simulink subsystem "As_Assembly"  (R2022b)
settings: Solver=VariableStepAuto  StartTime=0.0  StopTime=30  RelTol=1e-3
libraries: mbedblockslib x6, simulink x4, hdlsllib x2, slpidlib x2, fl_lib x1, nesl_utility x1
(part 3 of 3)

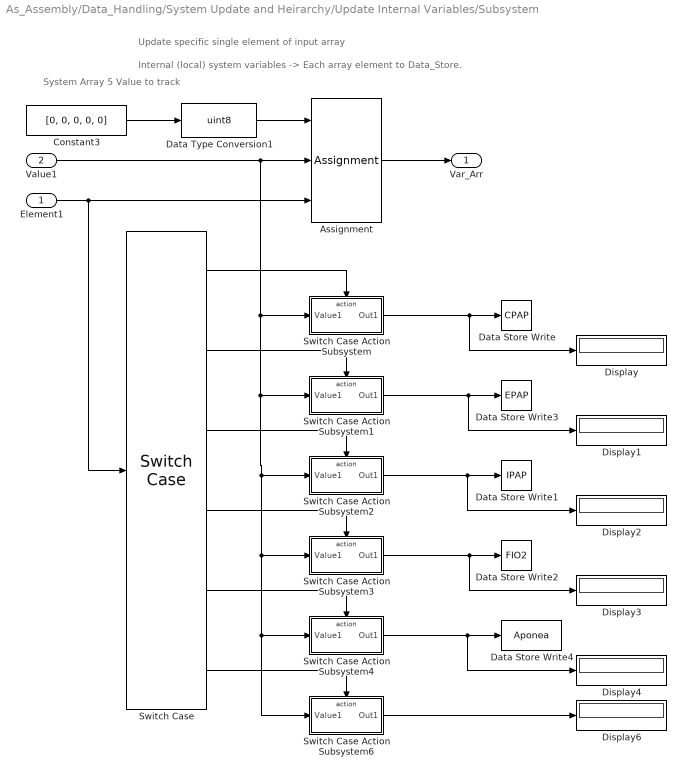
== system As_Assembly/Data_Handling/System Update and Heirarchy/Update Internal Variables/Subsystem ==
  note: System Array
      | 5 Value to track
  note: Update specific single element of input array
  note: Internal (local) system variables -> Each array element to Data_Store.
  Element1 : Inport
  Value1 : Inport  Port=2
  Assignment : Assignment  IndexMode=Zero-based  DiagnosticForDimensions=Warning  IndexOptions=Index vector (port)  Indices=0  OutputSizes=1
  Constant3 : Constant  Value=[0, 0, 0, 0, 0]
  Data Store Write : DataStoreWrite  DataStoreName=CPAP  IndexOptions=Index vector (dialog)  Indices=1  OutputSizes=1
  Data Store Write1 : DataStoreWrite  DataStoreName=IPAP  DataStoreElements=IPAP  IndexOptions=Index vector (dialog)  Indices=1  OutputSizes=1
  Data Store Write2 : DataStoreWrite  DataStoreName=FIO2  DataStoreElements=FIO2  IndexOptions=Index vector (dialog)  Indices=1  OutputSizes=1
  Data Store Write3 : DataStoreWrite  DataStoreName=EPAP  DataStoreElements=EPAP  IndexOptions=Index vector (dialog)  Indices=1  OutputSizes=1
  Data Store Write4 : DataStoreWrite  DataStoreName=Aponea  DataStoreElements=Aponea  IndexOptions=Index vector (dialog)  Indices=1  OutputSizes=1
  Data Type Conversion1 : DataTypeConversion  OutDataTypeStr=uint8  SaturateOnIntegerOverflow=off  RndMeth=Floor
  Display{,1..4,6} (6 alike) : Display
  Switch Case : SwitchCase  CaseConditions={0,1,2,3,4}
  Switch Case Action Subsystem : Subsystem  TreatAsAtomicUnit=on
  Switch Case Action Subsystem1 : Subsystem  TreatAsAtomicUnit=on
  Switch Case Action Subsystem2 : Subsystem  TreatAsAtomicUnit=on
  Switch Case Action Subsystem3 : Subsystem  TreatAsAtomicUnit=on
  Switch Case Action Subsystem4 : Subsystem  TreatAsAtomicUnit=on
  Switch Case Action Subsystem6 : Subsystem  TreatAsAtomicUnit=on
  Var_Arr : Outport
  wires:
  Switch Case/1 -> Switch Case Action Subsystem/Action
  Switch Case/3 -> Switch Case Action Subsystem2/Action
  Switch Case/2 -> Switch Case Action Subsystem1/Action
  Switch Case/4 -> Switch Case Action Subsystem3/Action
  Switch Case/6 -> Switch Case Action Subsystem6/Action
  Switch Case/5 -> Switch Case Action Subsystem4/Action
  Switch Case Action Subsystem6/1(Out1) -> Display6/1
  Switch Case Action Subsystem1/1(Out1) -> Display1/1, Data Store Write3/1
  Switch Case Action Subsystem2/1(Out1) -> Display2/1, Data Store Write1/1
  Switch Case Action Subsystem4/1(Out1) -> Display4/1, Data Store Write4/1
  Switch Case Action Subsystem3/1(Out1) -> Display3/1, Data Store Write2/1
  Value1/1 -> Assignment/2, Switch Case Action Subsystem/1(Value1), Switch Case Action Subsystem2/1(Value1), Switch Case Action Subsystem3/1(Value1), Switch Case Action Subsystem4/1(Value1), Switch Case Action Subsystem6/1(Value1), Switch Case Action Subsystem1/1(Value1)
  Switch Case Action Subsystem/1(Out1) -> Display/1, Data Store Write/1
  Assignment/1 -> Var_Arr/1
  Data Type Conversion1/1 -> Assignment/1
  Constant3/1 -> Data Type Conversion1/1
  Element1/1 -> Assignment/3, Switch Case/1

== system As_Assembly/Data_Handling/System Update and Heirarchy/Power_CMD/DC POWER/BAT: >25% ==
  In1 : Inport
  Action Port : ActionPort
  Out1 : Outport
  wires:
  In1/1 -> Out1/1

== system As_Assembly/Data_Handling/System Update and Heirarchy/Power_CMD/DC POWER/BAT: >75% ==
  In1 : Inport
  Action Port : ActionPort
  Out1 : Outport
  wires:
  In1/1 -> Out1/1

== system As_Assembly/Data_Handling/System Update and Heirarchy/Power_CMD/DC POWER/BAT:>50% ==
  In1 : Inport
  Action Port : ActionPort
  Out1 : Outport
  wires:
  In1/1 -> Out1/1

== system As_Assembly/Data_Handling/System Update and Heirarchy/Power_CMD/DC POWER/OUT OF RANGE ==
  In1 : Inport
  Action Port : ActionPort
  Out1 : Outport
  wires:
  In1/1 -> Out1/1

== system As_Assembly/Data_Handling/System Update and Heirarchy/Update Internal Variables/HMI_CMD1/ERROR MSG ==
  In1 : Inport
  Action Port : ActionPort
  Out1 : Outport
  wires:
  In1/1 -> Out1/1

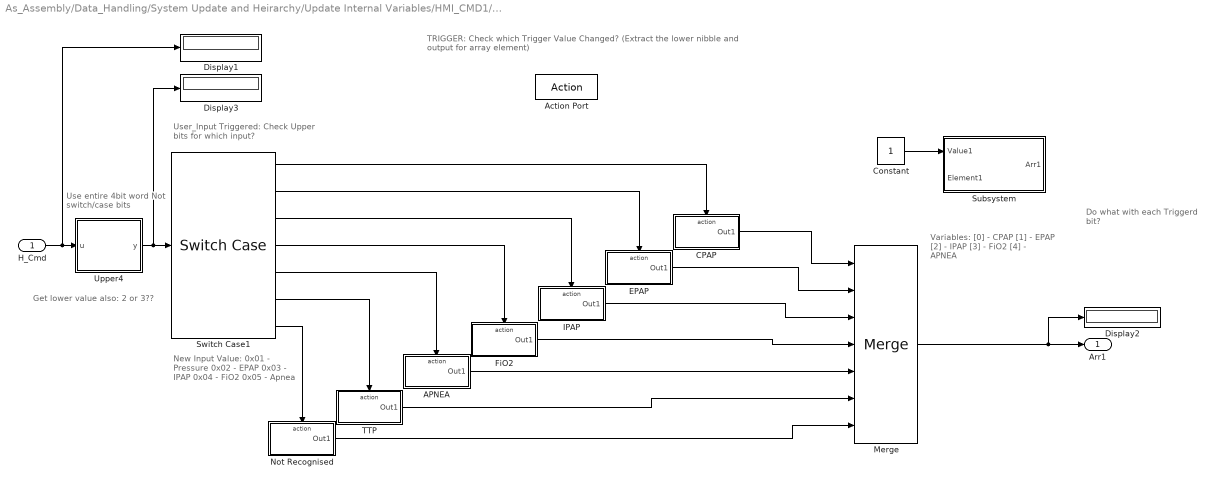
== system As_Assembly/Data_Handling/System Update and Heirarchy/Update Internal Variables/HMI_CMD1/EVENT TRGR ==
  note: TRIGGER: Check which Trigger Value Changed?
      | (Extract the lower nibble and output for array element)
  note: User_Input Triggered:
      | Check Upper bits for which input?
  note: Use entire 4bit word
      | Not switch/case bits
  note: Do what with each
      | Triggerd bit?
  note: New Input Value:
      | 0x01 - Pressure
      | 0x02 - EPAP
      | 0x03 - IPAP
      | 0x04 - FiO2
      | 0x05 - Apnea
  note: Get lower value also: 2 or 3??
  note: Variables:
      | [0] - CPAP
      | [1] - EPAP
      | [2] - IPAP
      | [3] - FiO2
      | [4] - APNEA
  H_Cmd : Inport
  Action Port : ActionPort
  APNEA : Subsystem  TreatAsAtomicUnit=on
  CPAP : Subsystem  TreatAsAtomicUnit=on
  Constant : Constant
  Display1 : Display
  Display2 : Display
  Display3 : Display
  EPAP : Subsystem  TreatAsAtomicUnit=on
  FiO2 : Subsystem  TreatAsAtomicUnit=on
  IPAP : Subsystem  TreatAsAtomicUnit=on
  Merge : Merge  Inputs=7
  Not Recognised : Subsystem  TreatAsAtomicUnit=on
  Subsystem : Subsystem
  Switch Case1 : SwitchCase  CaseConditions={0x00, 0x01, 0x02, 0x03, 0x04, 0x05}
  TTP : Subsystem  TreatAsAtomicUnit=on
  Upper4 : Subsystem
  Arr1 : Outport
  wires:
  Switch Case1/2 -> EPAP/Action
  Switch Case1/1 -> CPAP/Action
  Switch Case1/7 -> Not Recognised/Action
  CPAP/1(Out1) -> Merge/1
  EPAP/1(Out1) -> Merge/2
  Not Recognised/1(Out1) -> Merge/7
  Switch Case1/3 -> IPAP/Action
  Switch Case1/4 -> FiO2/Action
  IPAP/1(Out1) -> Merge/3
  FiO2/1(Out1) -> Merge/4
  H_Cmd/1 -> Display1/1, Upper4/1(u)
  Upper4/1(y) -> Display3/1, Switch Case1/1
  Constant/1 -> Subsystem/1(Value1)
  Switch Case1/5 -> APNEA/Action
  Switch Case1/6 -> TTP/Action
  Merge/1 -> Display2/1, Arr1/1
  APNEA/1(Out1) -> Merge/5
  TTP/1(Out1) -> Merge/6

== system As_Assembly/Data_Handling/System Update and Heirarchy/Update Internal Variables/HMI_CMD1/NO USER_IN ==
  note: No User_Input from HMI - Do nothing
      | Continue Normal Operation
  note: was arr[5]
  Action Port : ActionPort
  Constant5 : Constant  Value=0
  Out1 : Outport
  wires:
  Constant5/1 -> Out1/1

== system As_Assembly/Data_Handling/System Update and Heirarchy/Update Internal Variables/Subsystem/Switch Case Action Subsystem ==
  Value1 : Inport
  Action Port : ActionPort
  Out1 : Outport
  wires:
  Value1/1 -> Out1/1

== system As_Assembly/Data_Handling/System Update and Heirarchy/Update Internal Variables/Subsystem/Switch Case Action Subsystem1 ==
  Value1 : Inport
  Action Port : ActionPort
  Out1 : Outport
  wires:
  Value1/1 -> Out1/1

== system As_Assembly/Data_Handling/System Update and Heirarchy/Update Internal Variables/Subsystem/Switch Case Action Subsystem2 ==
  Value1 : Inport
  Action Port : ActionPort
  Out1 : Outport
  wires:
  Value1/1 -> Out1/1

== system As_Assembly/Data_Handling/System Update and Heirarchy/Update Internal Variables/Subsystem/Switch Case Action Subsystem3 ==
  Value1 : Inport
  Action Port : ActionPort
  Out1 : Outport
  wires:
  Value1/1 -> Out1/1

== system As_Assembly/Data_Handling/System Update and Heirarchy/Update Internal Variables/Subsystem/Switch Case Action Subsystem4 ==
  Value1 : Inport
  Action Port : ActionPort
  Out1 : Outport
  wires:
  Value1/1 -> Out1/1

== system As_Assembly/Data_Handling/System Update and Heirarchy/Update Internal Variables/Subsystem/Switch Case Action Subsystem6 ==
  Value1 : Inport
  Action Port : ActionPort
  Out1 : Outport
  wires:
  Value1/1 -> Out1/1

== system As_Assembly/Data_Handling/System Update and Heirarchy/Update Internal Variables/HMI_CMD1/EVENT TRGR/APNEA ==
  note: APNEA
  Action Port : ActionPort
  Constant : Constant  Value=4
  Out1 : Outport
  wires:
  Constant/1 -> Out1/1

== system As_Assembly/Data_Handling/System Update and Heirarchy/Update Internal Variables/HMI_CMD1/EVENT TRGR/CPAP ==
  Action Port : ActionPort
  Constant : Constant  Value=0
  Out1 : Outport
  wires:
  Constant/1 -> Out1/1

== system As_Assembly/Data_Handling/System Update and Heirarchy/Update Internal Variables/HMI_CMD1/EVENT TRGR/EPAP ==
  note: EPAP
  Action Port : ActionPort
  Constant : Constant
  Out1 : Outport
  wires:
  Constant/1 -> Out1/1

== system As_Assembly/Data_Handling/System Update and Heirarchy/Update Internal Variables/HMI_CMD1/EVENT TRGR/FiO2 ==
  note: FiO2
  Action Port : ActionPort
  Constant : Constant  Value=3
  Out1 : Outport
  wires:
  Constant/1 -> Out1/1

== system As_Assembly/Data_Handling/System Update and Heirarchy/Update Internal Variables/HMI_CMD1/EVENT TRGR/IPAP ==
  note: IPAP
  Action Port : ActionPort
  Constant : Constant  Value=2
  Out1 : Outport
  wires:
  Constant/1 -> Out1/1

== system As_Assembly/Data_Handling/System Update and Heirarchy/Update Internal Variables/HMI_CMD1/EVENT TRGR/Not Recognised ==
  note: Must be within array element range [0-3]
  Action Port : ActionPort
  Constant : Constant  Value=0
  Out1 : Outport
  wires:
  Constant/1 -> Out1/1

== system As_Assembly/Data_Handling/System Update and Heirarchy/Update Internal Variables/HMI_CMD1/EVENT TRGR/Subsystem ==
  note: Update single element of input array
  Value1 : Inport
  Element1 : Inport  Port=2
  Assignment : Assignment  IndexMode=Zero-based  DiagnosticForDimensions=Warning  IndexOptions=Index vector (port)  Indices=0  OutputSizes=1
  Constant5 : Constant  Value=[0,0,0,0]
  Arr1 : Outport
  wires:
  Constant5/1 -> Assignment/1
  Value1/1 -> Assignment/2
  Element1/1 -> Assignment/3
  Assignment/1 -> Arr1/1

== system As_Assembly/Data_Handling/System Update and Heirarchy/Update Internal Variables/HMI_CMD1/EVENT TRGR/TTP ==
  note: Time To Peak
  Action Port : ActionPort
  Constant : Constant  Value=5
  Out1 : Outport
  wires:
  Constant/1 -> Out1/1

== system As_Assembly/Data_Handling/System Update and Heirarchy/Update Internal Variables/HMI_CMD1/EVENT TRGR/Upper4 ==
  note: Get Upper 4 bits
  u : Inport
  Bit Shift1 : hdlsllib/Logic and Bit Operations/Bit Shift  mode=Shift Right Logical  N=4
  Data Type Conversion1 : DataTypeConversion  OutDataTypeStr=uint8  SaturateOnIntegerOverflow=off  RndMeth=Floor
  Extract Bits3 : simulink/Logic and Bit Operations/Extract Bits  bitsToExtract=Upper half  numBits=8  bitIdxRange=[0 7]  outScalingMode=Preserve fixed-point scaling
  y : Outport
  wires:
  Data Type Conversion1/1 -> Bit Shift1/1
  Bit Shift1/1 -> y/1
  Extract Bits3/1 -> Data Type Conversion1/1
  u/1 -> Extract Bits3/1

== stateflow chart As_Assembly/Data_Handling/Sub-Systems Read/Chart ==
  state IPAP
    entry:
    output = [35,20];
    during:
    %output = [3,20];
  state EPAP
    entry:
    output = [19,4];
    during:
  (default) -> IPAP
  IPAP -> EPAP
  data: output output

== stateflow chart As_Assembly/HMI_User_Inputs/Chart ==
  state IPAP_out
    entry:
    Output = IPAP;
    exit:
  state EPAP_out
    entry:
    Output = EPAP;
    exit:
  (default) -> IPAP_out
  EPAP_out -> IPAP_out : after(2.6,sec)
  IPAP_out -> EPAP_out : after(1.4,sec)
  data: IPAP data_store_memory; Output output; EPAP data_store_memory
